simulink model "sim2"  (R2023a)
settings: Solver=FixedStepAuto  StartTime=0.0  StopTime=0.001  FixedStep=dt  RelTol=dt
values from neighbouring files (symbols this model uses):
  C = 1*10^-6    (= 1e-06)    [Lab5k.m]
  f1 = 10    [Lab2.m]    (also in Lab5k.m = 439822.9717)
  L = 4*10^-6    (= 4e-06)    [Lab5k.m]
  R = 10    [Lab5k.m]
settings Model: Creator=khald  LastModifiedBy=khald

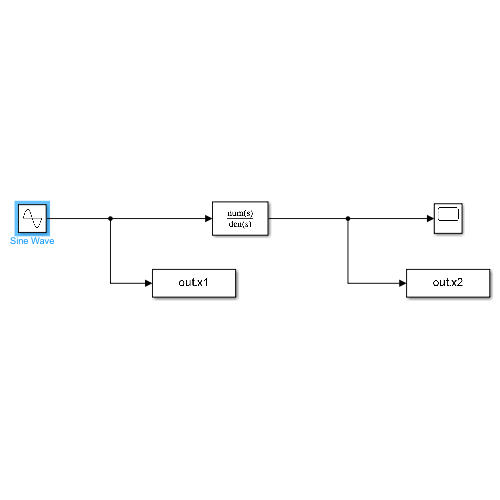
[thumbnail: Simulink's stored preview of the top-level diagram]
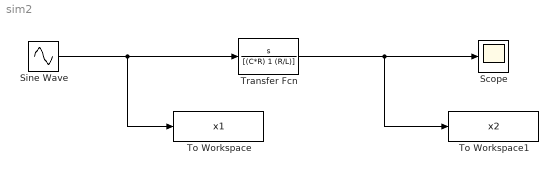
== system sim2 ==
  Scope : Scope
  Sine Wave : Sin  Frequency=f1  SampleTime=0
  To Workspace : ToWorkspace  VariableName=x1  SampleTime=-1
  To Workspace1 : ToWorkspace  VariableName=x2  SampleTime=-1
  Transfer Fcn : TransferFcn  Numerator=[1 0]  Denominator=[(C*R) 1 (R/L)]
  wires:
  Sine Wave/1 -> To Workspace/1, Transfer Fcn/1
  Transfer Fcn/1 -> To Workspace1/1, Scope/1
